simulink model "LQG"  (R2023a)
settings: Solver=VariableStepAuto  StartTime=0.0  StopTime=10.0  RelTol=1e-3
settings Model: Creator=belov  LastModifiedBy=belov

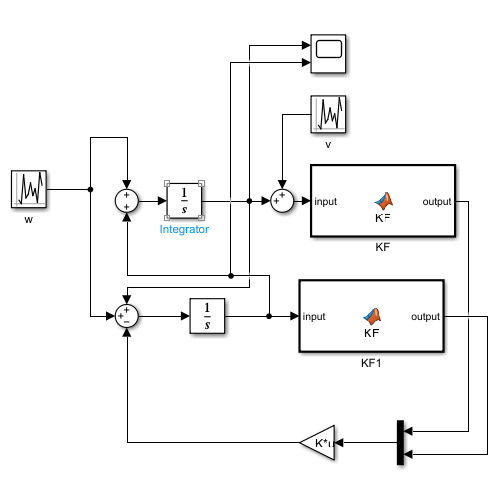
[thumbnail: Simulink's stored preview of the top-level diagram]
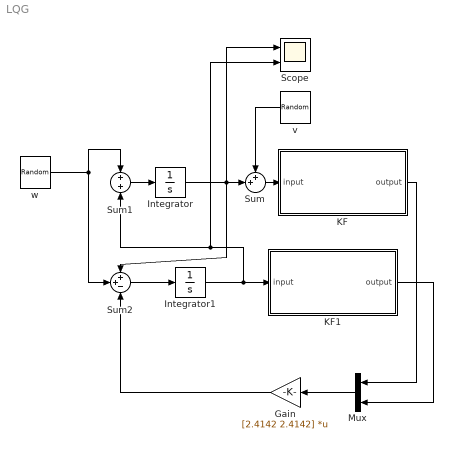
== system LQG ==
  Gain : Gain  Gain=[2.4142 2.4142]  Multiplication=Matrix(K*u)
  Integrator : Integrator  InitialCondition=1
  Integrator1 : Integrator  InitialCondition=1
  KF : MATLAB Function  TreatAsAtomicUnit=on  SystemSampleTime=0.001
  KF1 : MATLAB Function  TreatAsAtomicUnit=on  SystemSampleTime=0.001
  Mux : Mux  Inputs=2
  Scope : Scope  NumInputPorts=2
  Sum : Sum  Inputs=++|
  Sum1 : Sum  Inputs=+|+
  Sum2 : Sum  Inputs=++-
  v : UniformRandomNumber  Minimum=-0.05  Maximum=0.05  SampleTime=0.1
  w : UniformRandomNumber  Minimum=-0.05  Maximum=0.05  SampleTime=0.1
  wires:
  Sum/1 -> KF/1(input)
  v/1 -> Sum/1
  Integrator/1 -> Sum/2, Sum2/1, Scope/1
  Sum1/1 -> Integrator/1
  Sum2/1 -> Integrator1/1
  w/1 -> Sum1/1, Sum2/2
  KF/1(output) -> Mux/1
  Integrator1/1 -> KF1/1(input), Scope/2, Sum1/2
  Mux/1 -> Gain/1
  Gain/1 -> Sum2/3
  KF1/1(output) -> Mux/2

== matlab function LQG/KF ==
  data: input input; output output
function output = KF(input)
persistent x_last_last P_last_last;
if(isempty(x_last_last))
    x_last_last = 0;
end
if(isempty(P_last_last))
    P_last_last = 1;
end

F_k = 1;
H_k = 1;

Q_k = 1;
R_k = 4;



x_last_now = F_k * x_last_last;
P_last_now = F_k * P_last_last * F_k' + Q_k;
K_k = P_last_now * H_k' * inv(H_k * P_last_now * H_k' + R_k);
x_now_now = x_last_now + K_k * (input - H_k * x_last_now);
I = eye(size(K_k * H_k));
P_last_last = (I - K_k * H_k) * P_last_now;
x_last_last = x_now_now;

output = x_now_now;

== matlab function LQG/KF1 ==
  data: input input; output output
function output = KF(input)
persistent x_last_last P_last_last;
if(isempty(x_last_last))
    x_last_last = 0;
end
if(isempty(P_last_last))
    P_last_last = 1;
end

F_k = 1;
H_k = 1;

Q_k = 1;
R_k = 4;



x_last_now = F_k * x_last_last;
P_last_now = F_k * P_last_last * F_k' + Q_k;
K_k = P_last_now * H_k' * inv(H_k * P_last_now * H_k' + R_k);
x_now_now = x_last_now + K_k * (input - H_k * x_last_now);
I = eye(size(K_k * H_k));
P_last_last = (I - K_k * H_k) * P_last_now;
x_last_last = x_now_now;

output = x_now_now;
